simulink model "TerrainFollowing"  (Simulink 9.2)
settings: Solver=VariableStepAuto  StartTime=0.0  StopTime=60  RelTol=1e-3
values from neighbouring files (symbols this model uses):
  A_terrainfollow = A_temp(1:n_states,1:n_states)    [AE4301p.m]
  altitude0 = altitude0 * feet_to_m    [AE4301p.m]    (also in Settings.m = 15000)
  B_terrainfollow = A_temp(1:n_states,n_states+1:n_states+n_inputs)    [AE4301p.m]
  C_terrainfollow = C_temp(1:n_states,1:n_states)    [AE4301p.m]
  C_terrainfollow_inv = inv(C_terrainfollow)    [AE4301p.m]
  D_terrainfollow = C_temp(1:n_states,n_states+1:n_states+n_inputs)    [AE4301p.m]
  elevator0 = xu_lo(14)    [AE4301p.m]
  elevator_max = 25    [Settings.m]
  elevator_min = -25    [Settings.m]
  feet_to_m = 0.3048    [Settings.m]
  thrust0 = xu_lo(13)    [AE4301p.m]
  thrust_max = thrust_max*lbf_to_N    (= 84516.218)    [Settings.m]
  thrust_min = thrust_min*lbf_to_N    (= 4448.222)    [Settings.m]
  USE_SI_UNITS = 0    [Settings.m]
  UseOptimalControl = 1    [AE4301p.m]
  velocity0 = velocity0 * feet_to_m    [AE4301p.m]    (also in Settings.m = 500)
  x_terrainfollow0 = zeros(1,n_states)    [AE4301p.m]
undefined symbols (not defined in the file or in its folder): K
libraries: simulink x3
settings Model: Creator=Hyperion  LastModifiedBy=Hyperion
settings Model: SuppressorTable=|
  | <?xml version="1.0" encoding="UTF-8" standalone="yes" ?>
  | <!DOCTYPE boost_serialization>
  | <boost_serialization signature="serialization::archive" version="15">
  | <DiagnosticSuppressor class_id="0" tracking_level="0" version="6">
  | 	<Table class_id="1" tracking_level="0" version="0">
  | 		<count>1</count>
  | 		<bucket_count>8</bucket_count>
  | 		<item_version>0</item_version>
  | 		<item class_id="2" tracking_level="0" version="0">
  | 			<first class_id="3" tracking_level="0" version="6">
  | 				<Source class_id="4" tracking_level="0" version="0">
  | 					<count>1</count>
  | 					<item_version>0</item_version>
  | 					<item>TerrainFollowing/Cost Average</item>
  | 				</Source>
  | 			</first>
  | 			<second class_id="5" tracking_level="0" version="6">
  | 				<SuppressedData class_id="6" tracking_level="0" version="0">
  | 					<count>1</count>
  | 					<bucket_count>8</bucket_count>
  | 					<item_version>0</item_version>
  | 					<item class_id="7" tracking_level="0" version="0">
  | 						<first class_id="8" tracking_level="0" version="6">
  | 							<ID>Simulink:blocks:DivideByZero</ID>
  | 							<Cause>
  | 								<Source>
  | 									<count>0</count>
  | 									<item_version>0</item_version>
  | 								</Source>
  | 							</Cause>
  | 						</first>
  | 						<second class_id="9" tracking_level="0" version="6">
  | 							<Comment></Comment>
  | 							<User>Hyperion</User>
  | 							<LastModified class_id="10" tracking_level="0" version="0">
  | 								<ptime_date class_id="11" tracking_level="0" version="0">
  | 									<date>20181218</date>
  | 								</ptime_date>
  | 								<ptime_time_duration class_id="12" tracking_level="0" version="0">
  | 									<is_special>0</is_special>
  | 									<time_duration_hours>12</time_duration_hours>
  | 									<time_duration_minutes>11</time_duration_minutes>
  | 									<time_duration_seconds>56</time_duration_seconds>
  | 									<time_duration_fractional_seconds>0</time_duration_fractional_seconds>
  | 								</ptime_time_duration>
  | 							</LastModified>
  | 							<SuppressionType>0</SuppressionType>
  | 						</second>
  | 					</item>
  | 				</SuppressedData>
  | 			</second>
  | 		</item>
  | 	</Table>
  | </DiagnosticSuppressor>
  | </boost_serialization>
settings DataIOCC: LimitDataPoints=off  SaveFormat=Dataset  SignalLoggingSaveFormat=Dataset
settings OptimizationCC: LifeSpan=auto
settings DebuggingCC: UnderspecifiedInitializationDetection=Simplified  MergeDetectMultiDrivingBlocksExec=error  FcnCallInpInsideContextMsg=error  StateNameClashWarn=none  SFUnexpectedBacktrackingDiag=error  SFNoUnconditionalDefaultTransitionDiag=error  SFExecutionAtInitializationDiag=warning
settings HardwareCC: ProdBitPerPointer=64  ProdBitPerSizeT=64  ProdBitPerPtrDiffT=64  ProdLargestAtomicFloat=Float  ProdIntDivRoundTo=Zero  ProdEndianess=LittleEndian  ProdWordSize=64  ProdHWDeviceType=Intel->x86-64 (Windows64)
settings ModelReferenceCC: PropagateSignalLabelsOutOfModel=on
settings SFSimCC: SimUseLocalCustomCode=on
settings RTWCC: RTWUseLocalCustomCode=on
settings CodeAppCC: StateflowObjectComments=off
settings GRTTargetCC: TargetLangStandard=C99 (ISO)  GeneratePreprocessorConditionals=Use local settings  CombineOutputUpdateFcns=on  GRTInterface=off
settings ConfigComp: CovMetricSettings=dwe  CovHtmlReporting=off  CovSaveCumulativeToWorkspaceVar=off  CovSaveSingleToWorkspaceVar=off  CovExternalEMLEnable=on

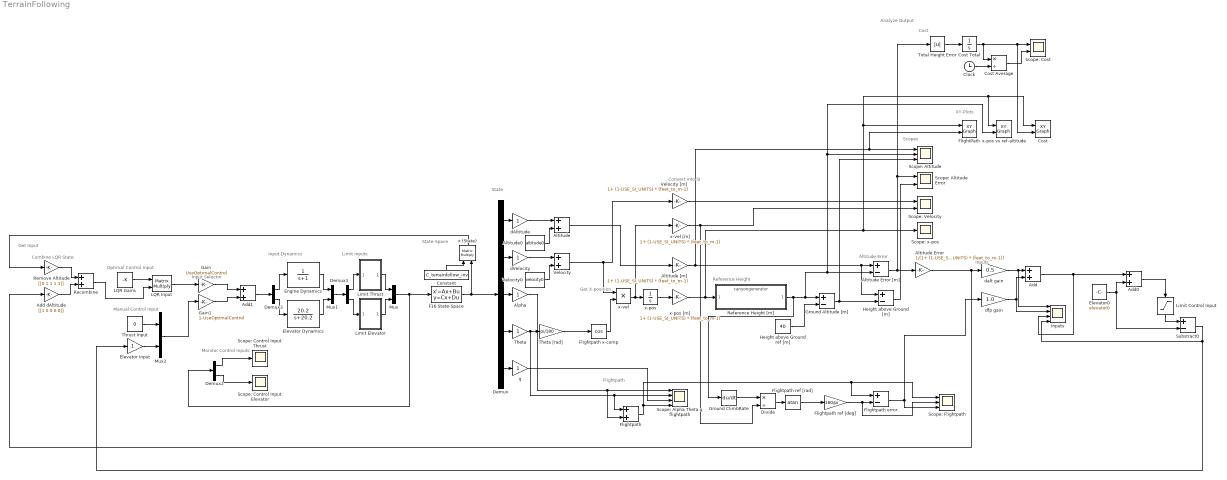
== system TerrainFollowing ==
  note: Combine LQR State
  note: State-Space
  note: Monitor Control Inputs
  note: Analyze Output
  note: Get Input
  note: Optimal Control Input
  note: Input Selector
  note: Altitude Error
  note: Convert into SI
  note: Get X-position
  note: State
  note: Reference Height
  note: XY-Plots
  note: Scopes
  note: Inputs
  note: Flightpath
  note: Manual Control Input
  note: Cost
  note: Limit Inputs
  note: Input Dynamics
  Add : Sum
  Add dAltitude : Gain  Gain=[[1 0 0 0 0]]
  Add0 : Sum
  Add1 : Sum
  Alpha : Gain
  Altitude : Sum
  Altitude Error : Gain  Gain=1/(1+ (1-USE_SI_UNITS) * (feet_to_m-1))
  Altitude Error [m] : Sum  Inputs=+-
  Altitude [m] : Gain  Gain=1+ (1-USE_SI_UNITS) * (feet_to_m-1)
  Altitude0 : Constant  Value=altitude0
  Clock : Clock
  Constant : Constant  Value=C_terrainfollow_inv
  Cost : simulink/Sinks/XY Graph  xmin=0  xmax=6000  ymin=0  ymax=1000  st=-1
  Cost Average : Product  Inputs=*/
  Cost Total : Integrator
  Demux : Demux  Outputs=5
  Demux1 : Demux  Outputs=2
  Demux2 : Demux  Outputs=2
  Demux3 : Demux  Outputs=2
  Divide : Product  Inputs=*/
  Elevator Dynamics : TransferFcn  Numerator=[20.2]  Denominator=[1 20.2]
  Elevator Input : Gain
  Elevator0 : Constant  Value=elevator0
  Engine Dynamics : TransferFcn  Denominator=[1 1]
  F16 State-Space : StateSpace  A=A_terrainfollow  B=B_terrainfollow  C=C_terrainfollow  D=D_terrainfollow  InitialCondition=x_terrainfollow0
  FlightPath : simulink/Sinks/XY Graph  xmin=0  xmax=6000  ymin=1000  ymax=2000  st=-1
  Flightpath : Sum
  Flightpath error : Sum  Inputs=+-
  Flightpath ref [deg] : Gain  Gain=180/pi
  Flightpath ref [rad] : Trigonometry  Operator=atan
  Flightpath x-comp : Trigonometry  Operator=cos
  Gain : Gain  Gain=UseOptimalControl
  Gain1 : Gain  Gain=1-UseOptimalControl
  Ground Altitude [m] : Sum  Inputs=+-
  Ground ClimbRate : Derivative
  Height above Ground [m] : Sum  Inputs=+-
  Height above Ground ref [m] : Constant  Value=40
  Inputs : Scope  NumInputPorts=4
  LQR Gains : Constant  Value=-K
  LQR Input : Product  Multiplication=Matrix(*)
  Limit Control Input : Saturate  UpperLimit=25  LowerLimit=-25
  Limit Elevator : Subsystem
  Limit Thrust : Subsystem
  Mux : Mux  Inputs=2
  Mux1 : Mux  Inputs=2
  Mux2 : Mux  Inputs=2
  Recombine : Sum
  Reference Height [m] : ModelReference  ModelNameDialog=canyongenerator.mdl  SimulationMode=Normal  ModelReferenceVersion=1.8
  Remove Altitude : Gain  Gain=[[0 1 1 1 1]]
  Scope: Alpha Theta q flightpath : Scope  NumInputPorts=4
  Scope: Altitude : Scope  NumInputPorts=3
  Scope: Altitude Error : Scope  NumInputPorts=2
  Scope: Control Input Elevator : Scope
  Scope: Control Input Thrust : Scope
  Scope: Cost : Scope  NumInputPorts=2
  Scope: Flightpath : Scope  NumInputPorts=3
  Scope: Velocity : Scope  NumInputPorts=2
  Scope: x-pos : Scope
  Substract0 : Sum  Inputs=+-
  Theta : Gain
  Theta [rad] : Gain  Gain=pi/180
  Thrust Input : Constant  Value=0
  Total Height Error : Abs
  Velocity : Sum
  Velocity [m] : Gain  Gain=1+ (1-USE_SI_UNITS) * (feet_to_m-1)
  Velocity0 : Constant  Value=velocity0
  dAltitude : Gain
  dVelocity : Gain
  dalt gain : Gain  Gain=0.5  OutMin=-25  OutMax=25
  dfp gain : Gain  Gain=1.0  OutMin=-25  OutMax=25
  q : Gain
  x (State) : Product  Multiplication=Matrix(*)
  x-pos : Integrator
  x-pos [m] : Gain  Gain=1+ (1-USE_SI_UNITS) * (feet_to_m-1)
  x-pos vs ref-altitude : simulink/Sinks/XY Graph  xmin=0  xmax=6000  ymin=1000  ymax=2000  st=-1
  x-vel : Product
  x-vel [m] : Gain  Gain=1+ (1-USE_SI_UNITS) * (feet_to_m-1)
  wires:
  Reference Height [m]/1 -> Ground Altitude [m]/1, Scope: Altitude/2, x-pos vs ref-altitude/2, Altitude Error [m]/2, Ground ClimbRate/1
  Altitude Error [m]/1 -> Altitude Error/1, Total Height Error/1, Scope: Altitude Error/1
  Thrust Input/1 -> Mux2/1
  F16 State-Space/1 -> Demux/1, x (State)/2
  Demux/2 -> dVelocity/1
  Demux/1 -> dAltitude/1
  dVelocity/1 -> Velocity/1
  Velocity0/1 -> Velocity/2
  Height above Ground ref [m]/1 -> Ground Altitude [m]/2
  Ground Altitude [m]/1 -> Height above Ground [m]/2, Scope: Altitude/3
  x-vel/1 -> x-vel [m]/1, x-pos/1
  Velocity/1 -> x-vel/1, Velocity [m]/1
  Flightpath x-comp/1 -> x-vel/2
  Demux/4 -> Theta/1
  Theta/1 -> Theta [rad]/1, Flightpath/1, Scope: Alpha Theta q flightpath/2
  Elevator Input/1 -> Mux2/2
  x-pos [m]/1 -> Reference Height [m]/1, x-pos vs ref-altitude/1, Cost/1, FlightPath/1, Scope: x-pos/1
  x-pos/1 -> x-pos [m]/1
  Altitude [m]/1 -> FlightPath/2, Scope: Altitude/1, Height above Ground [m]/1, Altitude Error [m]/1
  dAltitude/1 -> Altitude/1
  Altitude0/1 -> Altitude/2
  Altitude/1 -> Altitude [m]/1
  Altitude Error/1 -> Add dAltitude/1, dalt gain/1
  Demux/3 -> Alpha/1
  Alpha/1 -> Flightpath/2, Scope: Alpha Theta q flightpath/1
  Demux/5 -> q/1
  q/1 -> Scope: Alpha Theta q flightpath/3
  Theta [rad]/1 -> Flightpath x-comp/1
  dalt gain/1 -> Inputs/1, Add/1
  Add/1 -> Add0/1, Inputs/3
  dfp gain/1 -> Add/2, Inputs/2
  Ground ClimbRate/1 -> Divide/1
  Divide/1 -> Flightpath ref [rad]/1
  Velocity [m]/1 -> Scope: Velocity/1
  x-vel [m]/1 -> Divide/2, Scope: Velocity/2
  Flightpath/1 -> Scope: Flightpath/1, Flightpath error/1, Scope: Alpha Theta q flightpath/4
  Flightpath error/1 -> Scope: Flightpath/3, dfp gain/1
  Flightpath ref [rad]/1 -> Flightpath ref [deg]/1
  Flightpath ref [deg]/1 -> Scope: Flightpath/2, Flightpath error/2
  Total Height Error/1 -> Cost Total/1
  Cost Total/1 -> Cost Average/1, Scope: Cost/1, Cost/2
  Height above Ground [m]/1 -> Scope: Altitude Error/2
  Clock/1 -> Cost Average/2
  Cost Average/1 -> Scope: Cost/2
  Gain/1 -> Add1/1
  Gain1/1 -> Add1/2
  LQR Input/1 -> Gain/1
  Mux2/1 -> Gain1/1
  LQR Gains/1 -> LQR Input/1
  Add0/1 -> Limit Control Input/1
  Elevator0/1 -> Substract0/2, Add0/2
  Limit Control Input/1 -> Substract0/1
  Substract0/1 -> Elevator Input/1, Inputs/4
  Limit Thrust/1(Out1) -> Mux/1
  Limit Elevator/1(Out1) -> Mux/2
  Demux1/1 -> Limit Thrust/1(In1)
  Demux1/2 -> Limit Elevator/1(In1)
  Mux/1 -> F16 State-Space/1, Demux2/1
  Demux2/1 -> Scope: Control Input Thrust/1
  Demux2/2 -> Scope: Control Input Elevator/1
  Engine Dynamics/1 -> Mux1/1
  Demux3/2 -> Elevator Dynamics/1
  Elevator Dynamics/1 -> Mux1/2
  Demux3/1 -> Engine Dynamics/1
  Add1/1 -> Demux3/1
  Mux1/1 -> Demux1/1
  Remove Altitude/1 -> Recombine/1
  Recombine/1 -> LQR Input/2
  Add dAltitude/1 -> Recombine/2
  x (State)/1 -> Remove Altitude/1
  Constant/1 -> x (State)/1

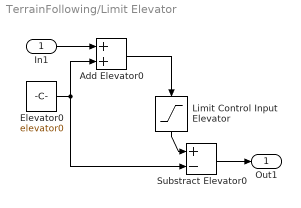
== system TerrainFollowing/Limit Elevator ==
  In1 : Inport
  Add Elevator0 : Sum
  Elevator0 : Constant  Value=elevator0
  Limit Control Input Elevator : Saturate  UpperLimit=elevator_max  LowerLimit=elevator_min
  Substract Elevator0 : Sum  Inputs=+-
  Out1 : Outport
  wires:
  Limit Control Input Elevator/1 -> Substract Elevator0/1
  Elevator0/1 -> Add Elevator0/2, Substract Elevator0/2
  In1/1 -> Add Elevator0/1
  Add Elevator0/1 -> Limit Control Input Elevator/1
  Substract Elevator0/1 -> Out1/1

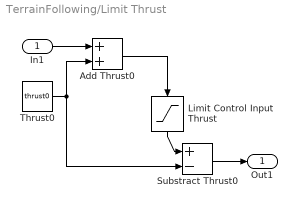
== system TerrainFollowing/Limit Thrust ==
  In1 : Inport
  Add Thrust0 : Sum
  Limit Control Input Thrust : Saturate  UpperLimit=thrust_max  LowerLimit=thrust_min
  Substract Thrust0 : Sum  Inputs=+-
  Thrust0 : Constant  Value=thrust0
  Out1 : Outport
  wires:
  Limit Control Input Thrust/1 -> Substract Thrust0/1
  Thrust0/1 -> Add Thrust0/2, Substract Thrust0/2
  In1/1 -> Add Thrust0/1
  Add Thrust0/1 -> Limit Control Input Thrust/1
  Substract Thrust0/1 -> Out1/1
